simulink model "CEngDsT_VDDynTst"  (R2016b)
settings: configuration reference "CodeGenConfigSet" (kept outside this file)
values from neighbouring files (symbols this model uses):
  CEngDsT_dtMinDynTst_CUR = Calibration.Parameter    [init_CEngDsT_VDDynTst.m]
  CEngDsT_dtMinDynTst_CURX = Calibration.Parameter    [init_CEngDsT_VDDynTst.m]
  CEngDsT_nMinEnaAbsTst_C = Calibration.Parameter    [init_CEngDsT_VDDynTst.m]
  CEngDsT_nMinEnaDynTst_C = Calibration.Parameter    [init_CEngDsT_VDDynTst.m]
  CEngDsT_qMinAbsTst_C = Calibration.Parameter    [init_CEngDsT_VDDynTst.m]
  CEngDsT_qMinEnaDynTst_C = Calibration.Parameter    [init_CEngDsT_VDDynTst.m]
  CEngDsT_tiIniTmr_C = Calibration.Parameter    [init_CEngDsT_VDDynTst.m]
  CEngDsT_tiMaxAbsTst_CUR = Calibration.Parameter    [init_CEngDsT_VDDynTst.m]
  CEngDsT_tiMaxAbsTst_CURX = Calibration.Parameter    [init_CEngDsT_VDDynTst.m]
  CEngDsT_tiMaxDynTst_CUR = Calibration.Parameter    [init_CEngDsT_VDDynTst.m]
  CEngDsT_tiMaxDynTst_CURX = Calibration.Parameter    [init_CEngDsT_VDDynTst.m]
  CEngDsT_tMinAbsTst_CUR = Calibration.Parameter    [init_CEngDsT_VDDynTst.m]
  CEngDsT_tMinAbsTst_CURX = Calibration.Parameter    [init_CEngDsT_VDDynTst.m]
  CEngDsT_tMinThresDynTst_C = Calibration.Parameter    [init_CEngDsT_VDDynTst.m]
undefined symbols (not defined in the file or in its folder): CEngDsT_tTransf_CURX, CEngDsT_VDDynTst_DT, EngState_conv
libraries: CXLib x5
settings Model: Creator=lenovo  LastModifiedBy=wangrui
settings ConfigSetRef: SourceLocation=Base Workspace

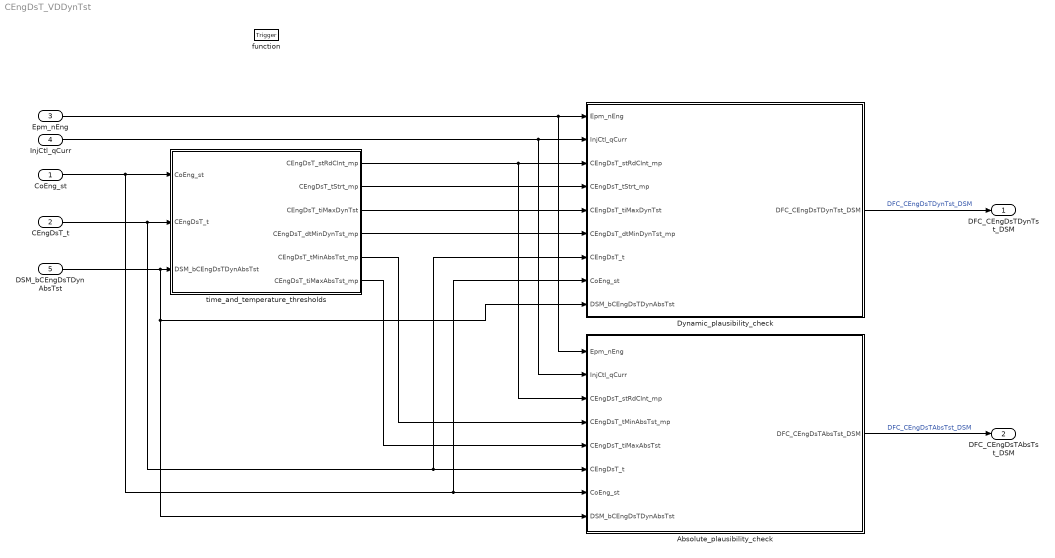
== system CEngDsT_VDDynTst ==
  CoEng_st : Inport  Description=Engine coordinator state  OutDataTypeStr=Enum: EngState_conv
  CEngDsT_t : Inport  Tag=deg  Description=engine coolant temperature after filter  Port=2  OutMin=-200  OutMax=200  OutDataTypeStr=Temp_deg
  Epm_nEng : Inport  Tag=rpm  Description=Engine speed  Port=3  OutMin=0  OutMax=6000  OutDataTypeStr=EngSpeed_rpm
  InjCtl_qCurr : Inport  Tag=mg/hub  Description=Torque generating engine fuel injection quantity  Port=4  OutMin=-319  OutMax=319  OutDataTypeStr=FuelMass_mg_hub
  DSM_bCEngDsTDynAbsTst : Inport  Description=state of FId_CEngDsTDynAbsTst  Port=5  OutMin=0  OutMax=1  OutDataTypeStr=boolean
  function : TriggerPort  TriggerType=function-call  VariantControl=Variant
  Absolute_plausibility_check : Subsystem  RequirementInfo={'other' 'CEngDsT_VDDynTst_requirements.doc' '@Simulink_requirement_item_3' 'true' '水温绝对值合理性校验' '' } %GIDa_49b2f334_2a18_42b0_a730_34b68f464cea
  Dynamic_plausibility_check : Subsystem  RequirementInfo={'other' 'CEngDsT_VDDynTst_requirements.doc' '@Simulink_requirement_item_2' 'true' '水温动态合理性校验' '' } %GIDa_29f8c977_1158_4d09_a78e_e4c79640a36b
  time_and_temperature_thresholds : Subsystem  RequirementInfo={'other' 'CEngDsT_VDDynTst_requirements.doc' '@Simulink_requirement_item_4' 'true' '水温动态和绝对值合理性校验参数计算' '' } %GIDa_436acdf0_f9c3_4326_aa51_de55f45c0a8d
  DFC_CEngDsTDynTst_DSM : Outport  Description=error state of DFC_CEngDsTDynTst  OutMin=0  OutMax=1  OutDataTypeStr=boolean
  DFC_CEngDsTAbsTst_DSM : Outport  Description=error state of DFC_CEngDsTAbsTst  Port=2  OutMin=0  OutMax=1  OutDataTypeStr=boolean
  wires:
  time_and_temperature_thresholds/3(CEngDsT_tiMaxDynTst) -> Dynamic_plausibility_check/5(CEngDsT_tiMaxDynTst)
  time_and_temperature_thresholds/6(CEngDsT_tiMaxAbsTst_mp) -> Absolute_plausibility_check/5(CEngDsT_tiMaxAbsTst)
  Epm_nEng/1 -> Absolute_plausibility_check/1(Epm_nEng), Dynamic_plausibility_check/1(Epm_nEng)
  time_and_temperature_thresholds/4(CEngDsT_dtMinDynTst_mp) -> Dynamic_plausibility_check/6(CEngDsT_dtMinDynTst_mp)
  time_and_temperature_thresholds/5(CEngDsT_tMinAbsTst_mp) -> Absolute_plausibility_check/4(CEngDsT_tMinAbsTst_mp)
  time_and_temperature_thresholds/1(CEngDsT_stRdClnt_mp) -> Absolute_plausibility_check/3(CEngDsT_stRdClnt_mp), Dynamic_plausibility_check/3(CEngDsT_stRdClnt_mp)
  InjCtl_qCurr/1 -> Absolute_plausibility_check/2(InjCtl_qCurr), Dynamic_plausibility_check/2(InjCtl_qCurr)
  time_and_temperature_thresholds/2(CEngDsT_tStrt_mp) -> Dynamic_plausibility_check/4(CEngDsT_tStrt_mp)
  CEngDsT_t/1 -> Dynamic_plausibility_check/7(CEngDsT_t), Absolute_plausibility_check/6(CEngDsT_t), time_and_temperature_thresholds/2(CEngDsT_t)
  CoEng_st/1 -> Dynamic_plausibility_check/8(CoEng_st), Absolute_plausibility_check/7(CoEng_st), time_and_temperature_thresholds/1(CoEng_st)
  DSM_bCEngDsTDynAbsTst/1 -> Absolute_plausibility_check/8(DSM_bCEngDsTDynAbsTst), Dynamic_plausibility_check/9(DSM_bCEngDsTDynAbsTst), time_and_temperature_thresholds/3(DSM_bCEngDsTDynAbsTst)
  Dynamic_plausibility_check/1(DFC_CEngDsTDynTst_DSM) -> DFC_CEngDsTDynTst_DSM/1  "DFC_CEngDsTDynTst_DSM"
  Absolute_plausibility_check/1(DFC_CEngDsTAbsTst_DSM) -> DFC_CEngDsTAbsTst_DSM/1  "DFC_CEngDsTAbsTst_DSM"

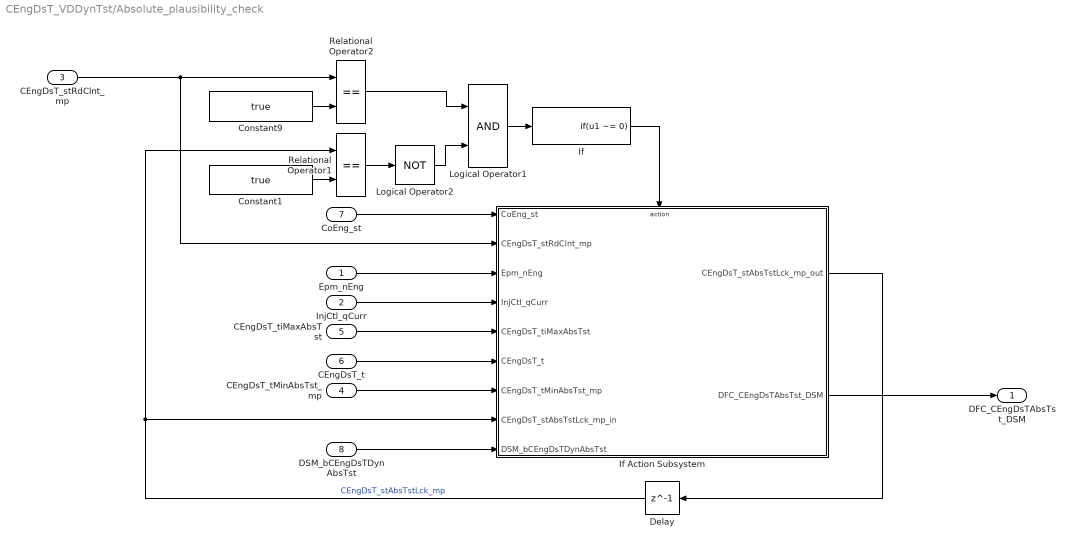
== system CEngDsT_VDDynTst/Absolute_plausibility_check ==
  Epm_nEng : Inport
  InjCtl_qCurr : Inport  Port=2
  CEngDsT_stRdClnt_mp : Inport  Port=3
  CEngDsT_tMinAbsTst_mp : Inport  Port=4
  CEngDsT_tiMaxAbsTst : Inport  Port=5
  CEngDsT_t : Inport  Port=6
  CoEng_st : Inport  Port=7
  DSM_bCEngDsTDynAbsTst : Inport  Description=state of FId_CEngDsTDynAbsTst  Port=8  OutMin=0  OutMax=1  OutDataTypeStr=boolean
  Constant1 : Constant  Value=true  VectorParams1D=off
  Constant9 : Constant  Value=true  VectorParams1D=off
  Delay : Delay  DelayLength=1  InitialCondition=0
  If : If  IfExpression=u1 ~= 0  ShowElse=off
  If Action Subsystem : Subsystem  TreatAsAtomicUnit=on
  Logical Operator1 : Logic  OutDataTypeStr=boolean
  Logical Operator2 : Logic  Operator=NOT  OutDataTypeStr=boolean
  Relational Operator1 : RelationalOperator  Operator===  OutDataTypeStr=boolean  RndMeth=Nearest  InputSameDT=on
  Relational Operator2 : RelationalOperator  Operator===  OutDataTypeStr=boolean  RndMeth=Nearest  InputSameDT=on
  DFC_CEngDsTAbsTst_DSM : Outport  Description=DFC_CEngDsTAbsTst  OutMin=0  OutMax=1  OutDataTypeStr=boolean
  wires:
  Delay/1 -> Relational Operator1/1, If Action Subsystem/8(CEngDsT_stAbsTstLck_mp_in)  "CEngDsT_stAbsTstLck_mp"
  If Action Subsystem/1(CEngDsT_stAbsTstLck_mp_out) -> Delay/1
  CEngDsT_stRdClnt_mp/1 -> If Action Subsystem/2(CEngDsT_stRdClnt_mp), Relational Operator2/1
  Constant9/1 -> Relational Operator2/2
  Constant1/1 -> Relational Operator1/2
  Relational Operator1/1 -> Logical Operator2/1
  Relational Operator2/1 -> Logical Operator1/1
  Logical Operator2/1 -> Logical Operator1/2
  Logical Operator1/1 -> If/1
  If/1 -> If Action Subsystem/Action
  CoEng_st/1 -> If Action Subsystem/1(CoEng_st)
  Epm_nEng/1 -> If Action Subsystem/3(Epm_nEng)
  InjCtl_qCurr/1 -> If Action Subsystem/4(InjCtl_qCurr)
  CEngDsT_tiMaxAbsTst/1 -> If Action Subsystem/5(CEngDsT_tiMaxAbsTst)
  CEngDsT_t/1 -> If Action Subsystem/6(CEngDsT_t)
  CEngDsT_tMinAbsTst_mp/1 -> If Action Subsystem/7(CEngDsT_tMinAbsTst_mp)
  DSM_bCEngDsTDynAbsTst/1 -> If Action Subsystem/9(DSM_bCEngDsTDynAbsTst)
  If Action Subsystem/2(DFC_CEngDsTAbsTst_DSM) -> DFC_CEngDsTAbsTst_DSM/1

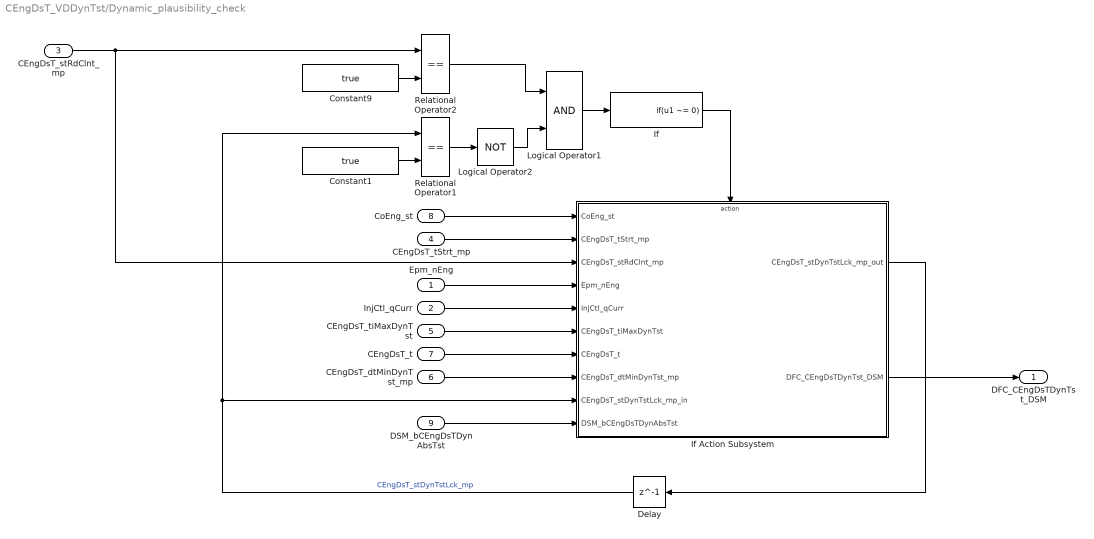
== system CEngDsT_VDDynTst/Dynamic_plausibility_check ==
  Epm_nEng : Inport
  InjCtl_qCurr : Inport  Port=2
  CEngDsT_stRdClnt_mp : Inport  Port=3
  CEngDsT_tStrt_mp : Inport  Port=4
  CEngDsT_tiMaxDynTst : Inport  Port=5
  CEngDsT_dtMinDynTst_mp : Inport  Port=6
  CEngDsT_t : Inport  Port=7
  CoEng_st : Inport  Port=8
  DSM_bCEngDsTDynAbsTst : Inport  Description=state of FId_CEngDsTDynAbsTst  Port=9  OutMin=0  OutMax=1  OutDataTypeStr=boolean
  Constant1 : Constant  Value=true  VectorParams1D=off
  Constant9 : Constant  Value=true  VectorParams1D=off
  Delay : Delay  DelayLength=1  InitialCondition=0
  If : If  IfExpression=u1 ~= 0  ShowElse=off
  If Action Subsystem : Subsystem  TreatAsAtomicUnit=on
  Logical Operator1 : Logic  OutDataTypeStr=boolean
  Logical Operator2 : Logic  Operator=NOT  OutDataTypeStr=boolean
  Relational Operator1 : RelationalOperator  Operator===  OutDataTypeStr=boolean  RndMeth=Nearest  InputSameDT=on
  Relational Operator2 : RelationalOperator  Operator===  OutDataTypeStr=boolean  RndMeth=Nearest  InputSameDT=on
  DFC_CEngDsTDynTst_DSM : Outport  Description=DFC_CEngDsTDynTst  OutMin=0  OutMax=1  OutDataTypeStr=boolean
  wires:
  CEngDsT_stRdClnt_mp/1 -> If Action Subsystem/3(CEngDsT_stRdClnt_mp), Relational Operator2/1
  Constant9/1 -> Relational Operator2/2
  Constant1/1 -> Relational Operator1/2
  Relational Operator1/1 -> Logical Operator2/1
  Relational Operator2/1 -> Logical Operator1/1
  Logical Operator2/1 -> Logical Operator1/2
  Logical Operator1/1 -> If/1
  If/1 -> If Action Subsystem/Action
  CEngDsT_tStrt_mp/1 -> If Action Subsystem/2(CEngDsT_tStrt_mp)
  CoEng_st/1 -> If Action Subsystem/1(CoEng_st)
  Epm_nEng/1 -> If Action Subsystem/4(Epm_nEng)
  InjCtl_qCurr/1 -> If Action Subsystem/5(InjCtl_qCurr)
  CEngDsT_tiMaxDynTst/1 -> If Action Subsystem/6(CEngDsT_tiMaxDynTst)
  CEngDsT_t/1 -> If Action Subsystem/7(CEngDsT_t)
  CEngDsT_dtMinDynTst_mp/1 -> If Action Subsystem/8(CEngDsT_dtMinDynTst_mp)
  If Action Subsystem/1(CEngDsT_stDynTstLck_mp_out) -> Delay/1
  Delay/1 -> If Action Subsystem/9(CEngDsT_stDynTstLck_mp_in), Relational Operator1/1  "CEngDsT_stDynTstLck_mp"
  DSM_bCEngDsTDynAbsTst/1 -> If Action Subsystem/10(DSM_bCEngDsTDynAbsTst)
  If Action Subsystem/2(DFC_CEngDsTDynTst_DSM) -> DFC_CEngDsTDynTst_DSM/1

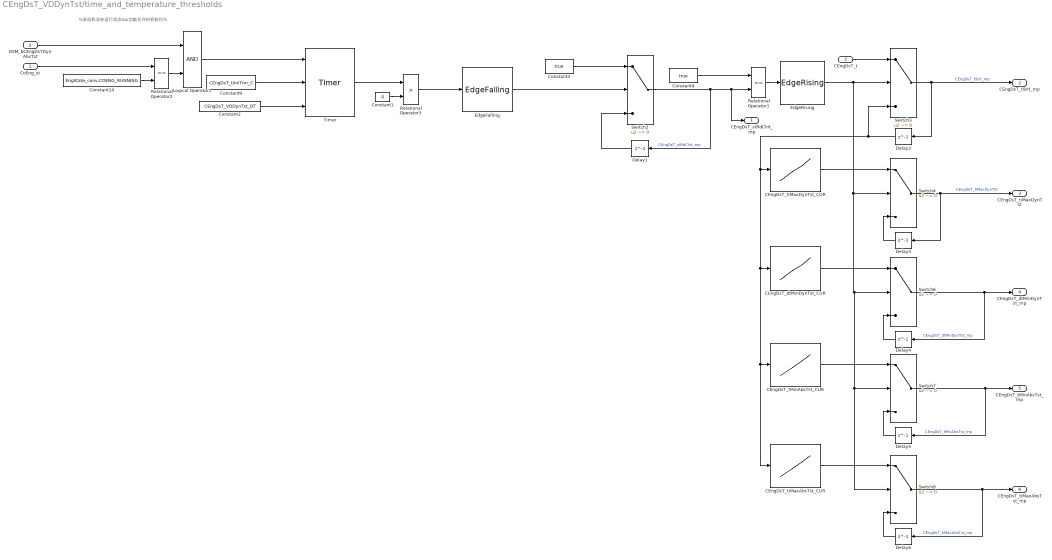
== system CEngDsT_VDDynTst/time_and_temperature_thresholds ==
  note: %发动机没在运行状态&&功能允许时初始化%
  CoEng_st : Inport
  CEngDsT_t : Inport  Port=2
  DSM_bCEngDsTDynAbsTst : Inport  Description=state of FId_CEngDsTDynAbsTst  Port=3  OutMin=0  OutMax=1  OutDataTypeStr=boolean
  CEngDsT_dtMinDynTst_CUR : Lookup_n-D  RequirementInfo={} %GIDa_f24a67d9_9be2_4f6a_98ff_fe8f3fd3d277  DialogController=Simulink.DDGSource  NumberOfTableDimensions=1  BreakpointsForDimension1=CEngDsT_dtMinDynTst_CURX  BreakpointsForDimension2=CEngDsT_tTransf_CURX  IndexSearchMethod=Linear search  BeginIndexSearchUsingPreviousIndexResult=on  Table=CEngDsT_dtMinDynTst_CUR  ExtrapMethod=Clip  UseLastTableValue=on  InternalRulePriority=Speed  OutDataTypeStr=Inherit: Inherit via back propagation  SaturateOnIntegerOverflow=on
  CEngDsT_tMinAbsTst_CUR : Lookup_n-D  RequirementInfo={} %GIDa_4fad5bf1_d5b2_4c41_9458_478ef92ce2f7  DialogController=Simulink.DDGSource  NumberOfTableDimensions=1  BreakpointsForDimension1=CEngDsT_tMinAbsTst_CURX  BreakpointsForDimension2=CEngDsT_tTransf_CURX  IndexSearchMethod=Linear search  BeginIndexSearchUsingPreviousIndexResult=on  Table=CEngDsT_tMinAbsTst_CUR  ExtrapMethod=Clip  UseLastTableValue=on  InternalRulePriority=Speed  OutDataTypeStr=Inherit: Inherit via back propagation  SaturateOnIntegerOverflow=on
  CEngDsT_tiMaxAbsTst_CUR : Lookup_n-D  RequirementInfo={} %GIDa_a4742909_2b6b_42c2_a6c4_82cb15b8cfec  DialogController=Simulink.DDGSource  NumberOfTableDimensions=1  BreakpointsForDimension1=CEngDsT_tiMaxAbsTst_CURX  BreakpointsForDimension2=CEngDsT_tTransf_CURX  IndexSearchMethod=Linear search  BeginIndexSearchUsingPreviousIndexResult=on  Table=CEngDsT_tiMaxAbsTst_CUR  ExtrapMethod=Clip  UseLastTableValue=on  InternalRulePriority=Speed  OutDataTypeStr=Inherit: Inherit via back propagation  SaturateOnIntegerOverflow=on
  CEngDsT_tiMaxDynTst_CUR : Lookup_n-D  RequirementInfo={} %GIDa_6227b4c9_a2a8_447e_8369_cb7c2ded31b1  DialogController=Simulink.DDGSource  NumberOfTableDimensions=1  BreakpointsForDimension1=CEngDsT_tiMaxDynTst_CURX  BreakpointsForDimension2=CEngDsT_tTransf_CURX  IndexSearchMethod=Linear search  BeginIndexSearchUsingPreviousIndexResult=on  Table=CEngDsT_tiMaxDynTst_CUR  ExtrapMethod=Clip  UseLastTableValue=on  InternalRulePriority=Speed  OutDataTypeStr=Inherit: Inherit via back propagation  SaturateOnIntegerOverflow=on
  Constant1 : Constant  Value=0  VectorParams1D=off  OutDataTypeStr=Inherit: Inherit via back propagation
  Constant14 : Constant  Value=EngState_conv.COENG_RUNNING
  Constant2 : Constant  Value=CEngDsT_VDDynTst_DT  VectorParams1D=off  OutDataTypeStr=Inherit: Inherit via back propagation
  Constant3 : Constant  Value=true  VectorParams1D=off  OutDataTypeStr=boolean
  Constant4 : Constant  Value=true  VectorParams1D=off  OutDataTypeStr=boolean
  Constant9 : Constant  Value=CEngDsT_tiIniTmr_C  VectorParams1D=off
  Delay{1..6} (6 alike) : Delay  DialogController=Simulink.DDGSource  DelayLength=1  InitialCondition=0
  EdgeFalling : CXLib/EdgeFalling
  EdgeRising : CXLib/EdgeRising
  Logical Operator1 : Logic  OutDataTypeStr=boolean
  Relational Operator1 : RelationalOperator  Operator===  OutDataTypeStr=boolean  RndMeth=Nearest  InputSameDT=on
  Relational Operator2 : RelationalOperator  Operator===  OutDataTypeStr=boolean  RndMeth=Nearest  InputSameDT=on
  Relational Operator3 : RelationalOperator  Operator=>  OutDataTypeStr=boolean  RndMeth=Nearest  InputSameDT=on
  Switch{2..4,6..8} (6 alike) : Switch  Criteria=u2 ~= 0  InputSameDT=on
  Timer : CXLib/Timer
  CEngDsT_stRdClnt_mp : Outport
  CEngDsT_tStrt_mp : Outport  Port=2
  CEngDsT_tiMaxDynTst : Outport  Port=3
  CEngDsT_dtMinDynTst_mp : Outport  Port=4
  CEngDsT_tMinAbsTst_mp : Outport  Port=5
  CEngDsT_tiMaxAbsTst_mp : Outport  Port=6
  wires:
  Constant2/1 -> Timer/3
  Relational Operator3/1 -> EdgeFalling/1
  Constant1/1 -> Relational Operator3/2
  Timer/1 -> Relational Operator3/1
  Constant9/1 -> Timer/2
  CEngDsT_tiMaxDynTst_CUR/1 -> Switch4/1
  Delay2/1 -> Switch3/3, CEngDsT_tiMaxAbsTst_CUR/1, CEngDsT_tMinAbsTst_CUR/1, CEngDsT_dtMinDynTst_CUR/1, CEngDsT_tiMaxDynTst_CUR/1
  Switch3/1 -> CEngDsT_tStrt_mp/1, Delay2/1  "CEngDsT_tStrt_mp"
  CEngDsT_t/1 -> Switch3/1
  EdgeRising/1 -> Switch3/2, Switch4/2, Switch6/2, Switch7/2, Switch8/2
  Relational Operator1/1 -> EdgeRising/1
  Constant4/1 -> Relational Operator1/1
  Delay1/1 -> Switch2/3
  Switch2/1 -> Delay1/1, Relational Operator1/2, CEngDsT_stRdClnt_mp/1  "CEngDsT_stRdClnt_mp"
  Constant3/1 -> Switch2/1
  EdgeFalling/1 -> Switch2/2
  Logical Operator1/1 -> Timer/1
  Relational Operator2/1 -> Logical Operator1/2
  DSM_bCEngDsTDynAbsTst/1 -> Logical Operator1/1
  CoEng_st/1 -> Relational Operator2/1
  Constant14/1 -> Relational Operator2/2
  Delay3/1 -> Switch4/3
  CEngDsT_tiMaxAbsTst_CUR/1 -> Switch8/1
  CEngDsT_tMinAbsTst_CUR/1 -> Switch7/1
  Switch7/1 -> CEngDsT_tMinAbsTst_mp/1, Delay5/1  "CEngDsT_tMinAbsTst_mp"
  Delay6/1 -> Switch8/3
  Delay5/1 -> Switch7/3
  Delay4/1 -> Switch6/3
  Switch8/1 -> Delay6/1, CEngDsT_tiMaxAbsTst_mp/1  "CEngDsT_tiMaxAbsTst_mp"
  CEngDsT_dtMinDynTst_CUR/1 -> Switch6/1
  Switch6/1 -> Delay4/1, CEngDsT_dtMinDynTst_mp/1  "CEngDsT_dtMinDynTst_mp"
  Switch4/1 -> Delay3/1, CEngDsT_tiMaxDynTst/1  "CEngDsT_tiMaxDynTst"

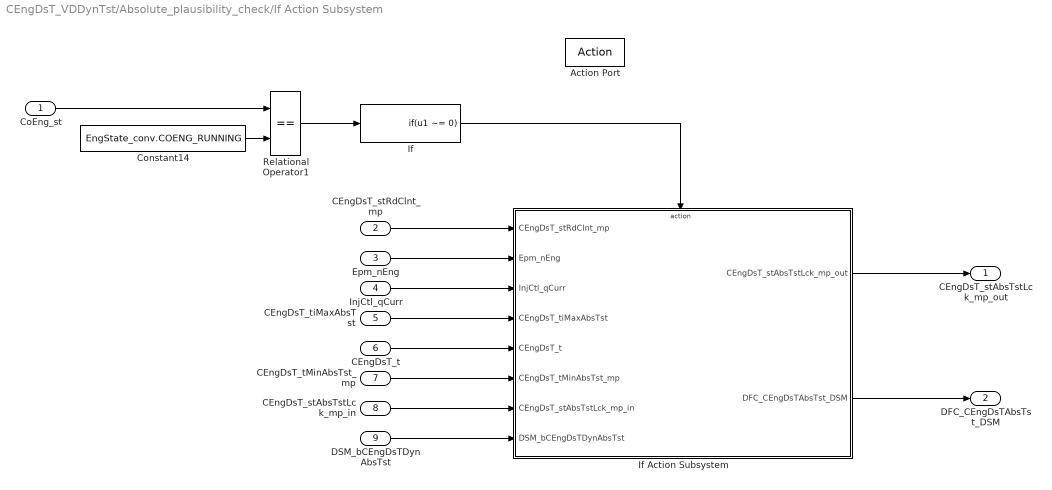
== system CEngDsT_VDDynTst/Absolute_plausibility_check/If Action Subsystem ==
  CoEng_st : Inport
  CEngDsT_stRdClnt_mp : Inport  Port=2
  Epm_nEng : Inport  Port=3
  InjCtl_qCurr : Inport  Port=4
  CEngDsT_tiMaxAbsTst : Inport  Port=5
  CEngDsT_t : Inport  Port=6
  CEngDsT_tMinAbsTst_mp : Inport  Port=7
  CEngDsT_stAbsTstLck_mp_in : Inport  Port=8
  DSM_bCEngDsTDynAbsTst : Inport  Description=state of FId_CEngDsTDynAbsTst  Port=9  OutMin=0  OutMax=1  OutDataTypeStr=boolean
  Action Port : ActionPort
  Constant14 : Constant  Value=EngState_conv.COENG_RUNNING
  If : If  IfExpression=u1 ~= 0  ShowElse=off
  If Action Subsystem : Subsystem  TreatAsAtomicUnit=on
  Relational Operator1 : RelationalOperator  Operator===  OutDataTypeStr=boolean  RndMeth=Nearest  InputSameDT=on
  CEngDsT_stAbsTstLck_mp_out : Outport
  DFC_CEngDsTAbsTst_DSM : Outport  Description=DFC_CEngDsTAbsTst  Port=2  OutMin=0  OutMax=1  OutDataTypeStr=boolean
  wires:
  If/1 -> If Action Subsystem/Action
  CoEng_st/1 -> Relational Operator1/1
  Constant14/1 -> Relational Operator1/2
  Relational Operator1/1 -> If/1
  If Action Subsystem/1(CEngDsT_stAbsTstLck_mp_out) -> CEngDsT_stAbsTstLck_mp_out/1
  CEngDsT_stRdClnt_mp/1 -> If Action Subsystem/1(CEngDsT_stRdClnt_mp)
  Epm_nEng/1 -> If Action Subsystem/2(Epm_nEng)
  InjCtl_qCurr/1 -> If Action Subsystem/3(InjCtl_qCurr)
  CEngDsT_tiMaxAbsTst/1 -> If Action Subsystem/4(CEngDsT_tiMaxAbsTst)
  CEngDsT_t/1 -> If Action Subsystem/5(CEngDsT_t)
  CEngDsT_tMinAbsTst_mp/1 -> If Action Subsystem/6(CEngDsT_tMinAbsTst_mp)
  CEngDsT_stAbsTstLck_mp_in/1 -> If Action Subsystem/7(CEngDsT_stAbsTstLck_mp_in)
  DSM_bCEngDsTDynAbsTst/1 -> If Action Subsystem/8(DSM_bCEngDsTDynAbsTst)
  If Action Subsystem/2(DFC_CEngDsTAbsTst_DSM) -> DFC_CEngDsTAbsTst_DSM/1

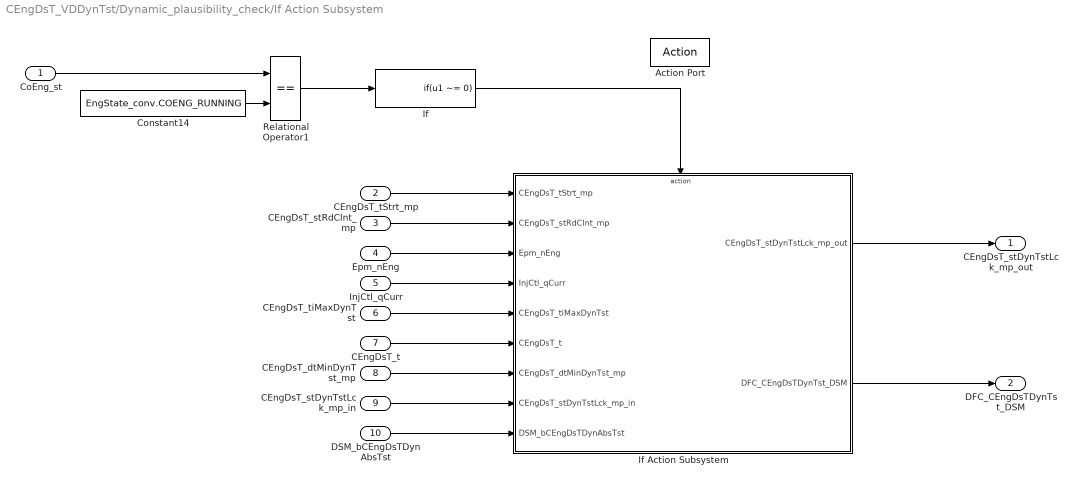
== system CEngDsT_VDDynTst/Dynamic_plausibility_check/If Action Subsystem ==
  CoEng_st : Inport
  CEngDsT_tStrt_mp : Inport  Port=2
  CEngDsT_stRdClnt_mp : Inport  Port=3
  Epm_nEng : Inport  Port=4
  InjCtl_qCurr : Inport  Port=5
  CEngDsT_tiMaxDynTst : Inport  Port=6
  CEngDsT_t : Inport  Port=7
  CEngDsT_dtMinDynTst_mp : Inport  Port=8
  CEngDsT_stDynTstLck_mp_in : Inport  Port=9
  DSM_bCEngDsTDynAbsTst : Inport  Description=state of FId_CEngDsTDynAbsTst  Port=10  OutMin=0  OutMax=1  OutDataTypeStr=boolean
  Action Port : ActionPort
  Constant14 : Constant  Value=EngState_conv.COENG_RUNNING
  If : If  IfExpression=u1 ~= 0  ShowElse=off
  If Action Subsystem : Subsystem  TreatAsAtomicUnit=on
  Relational Operator1 : RelationalOperator  Operator===  OutDataTypeStr=boolean  RndMeth=Nearest  InputSameDT=on
  CEngDsT_stDynTstLck_mp_out : Outport
  DFC_CEngDsTDynTst_DSM : Outport  Description=DFC_CEngDsTDynTst  Port=2  OutMin=0  OutMax=1  OutDataTypeStr=boolean
  wires:
  If/1 -> If Action Subsystem/Action
  CoEng_st/1 -> Relational Operator1/1
  Constant14/1 -> Relational Operator1/2
  Relational Operator1/1 -> If/1
  If Action Subsystem/1(CEngDsT_stDynTstLck_mp_out) -> CEngDsT_stDynTstLck_mp_out/1
  CEngDsT_stRdClnt_mp/1 -> If Action Subsystem/2(CEngDsT_stRdClnt_mp)
  Epm_nEng/1 -> If Action Subsystem/3(Epm_nEng)
  InjCtl_qCurr/1 -> If Action Subsystem/4(InjCtl_qCurr)
  CEngDsT_tStrt_mp/1 -> If Action Subsystem/1(CEngDsT_tStrt_mp)
  CEngDsT_tiMaxDynTst/1 -> If Action Subsystem/5(CEngDsT_tiMaxDynTst)
  CEngDsT_t/1 -> If Action Subsystem/6(CEngDsT_t)
  CEngDsT_dtMinDynTst_mp/1 -> If Action Subsystem/7(CEngDsT_dtMinDynTst_mp)
  CEngDsT_stDynTstLck_mp_in/1 -> If Action Subsystem/8(CEngDsT_stDynTstLck_mp_in)
  DSM_bCEngDsTDynAbsTst/1 -> If Action Subsystem/9(DSM_bCEngDsTDynAbsTst)
  If Action Subsystem/2(DFC_CEngDsTDynTst_DSM) -> DFC_CEngDsTDynTst_DSM/1

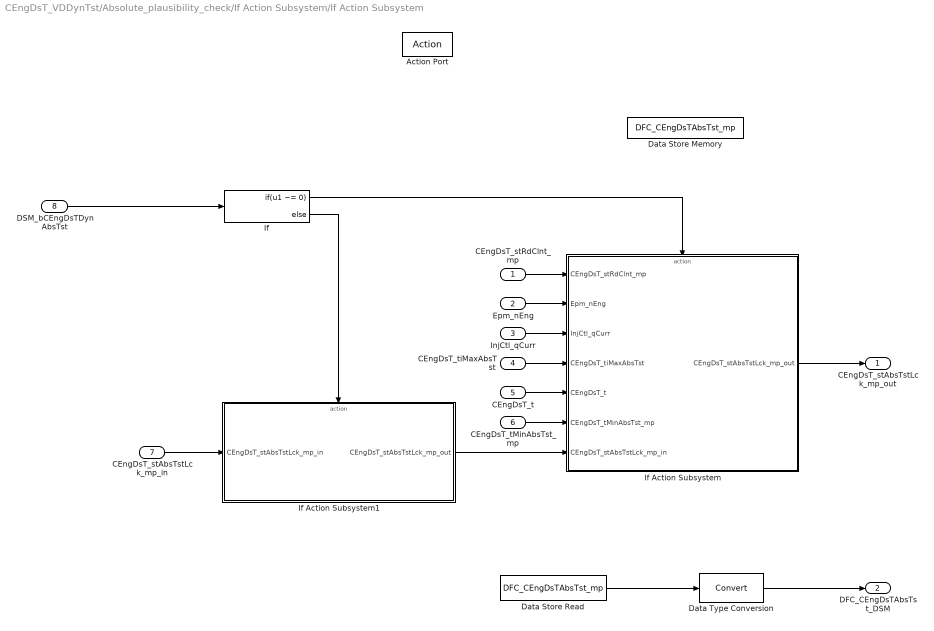
== system CEngDsT_VDDynTst/Absolute_plausibility_check/If Action Subsystem/If Action Subsystem ==
  CEngDsT_stRdClnt_mp : Inport
  Epm_nEng : Inport  Port=2
  InjCtl_qCurr : Inport  Port=3
  CEngDsT_tiMaxAbsTst : Inport  Port=4
  CEngDsT_t : Inport  Port=5
  CEngDsT_tMinAbsTst_mp : Inport  Port=6
  CEngDsT_stAbsTstLck_mp_in : Inport  Port=7
  DSM_bCEngDsTDynAbsTst : Inport  Description=state of FId_CEngDsTDynAbsTst  Port=8  OutMin=0  OutMax=1  OutDataTypeStr=boolean
  Action Port : ActionPort
  Data Store Memory : DataStoreMemory  DataStoreName=DFC_CEngDsTAbsTst_mp  ReadBeforeWriteMsg=warning  WriteAfterWriteMsg=warning  WriteAfterReadMsg=warning  ShowAdditionalParam=off
  Data Store Read : DataStoreRead  DataStoreName=DFC_CEngDsTAbsTst_mp
  Data Type Conversion : DataTypeConversion
  If : If  IfExpression=u1 ~= 0
  If Action Subsystem : Subsystem  TreatAsAtomicUnit=on
  If Action Subsystem1 : Subsystem  TreatAsAtomicUnit=on
  CEngDsT_stAbsTstLck_mp_out : Outport
  DFC_CEngDsTAbsTst_DSM : Outport  Description=DFC_CEngDsTAbsTst  Port=2  OutMin=0  OutMax=1  OutDataTypeStr=boolean
  wires:
  DSM_bCEngDsTDynAbsTst/1 -> If/1
  If/1 -> If Action Subsystem/Action
  If/2 -> If Action Subsystem1/Action
  If Action Subsystem1/1(CEngDsT_stAbsTstLck_mp_out) -> If Action Subsystem/7(CEngDsT_stAbsTstLck_mp_in)
  CEngDsT_stRdClnt_mp/1 -> If Action Subsystem/1(CEngDsT_stRdClnt_mp)
  If Action Subsystem/1(CEngDsT_stAbsTstLck_mp_out) -> CEngDsT_stAbsTstLck_mp_out/1
  CEngDsT_stAbsTstLck_mp_in/1 -> If Action Subsystem1/1(CEngDsT_stAbsTstLck_mp_in)
  Epm_nEng/1 -> If Action Subsystem/2(Epm_nEng)
  CEngDsT_tiMaxAbsTst/1 -> If Action Subsystem/4(CEngDsT_tiMaxAbsTst)
  InjCtl_qCurr/1 -> If Action Subsystem/3(InjCtl_qCurr)
  CEngDsT_t/1 -> If Action Subsystem/5(CEngDsT_t)
  CEngDsT_tMinAbsTst_mp/1 -> If Action Subsystem/6(CEngDsT_tMinAbsTst_mp)
  Data Store Read/1 -> Data Type Conversion/1
  Data Type Conversion/1 -> DFC_CEngDsTAbsTst_DSM/1

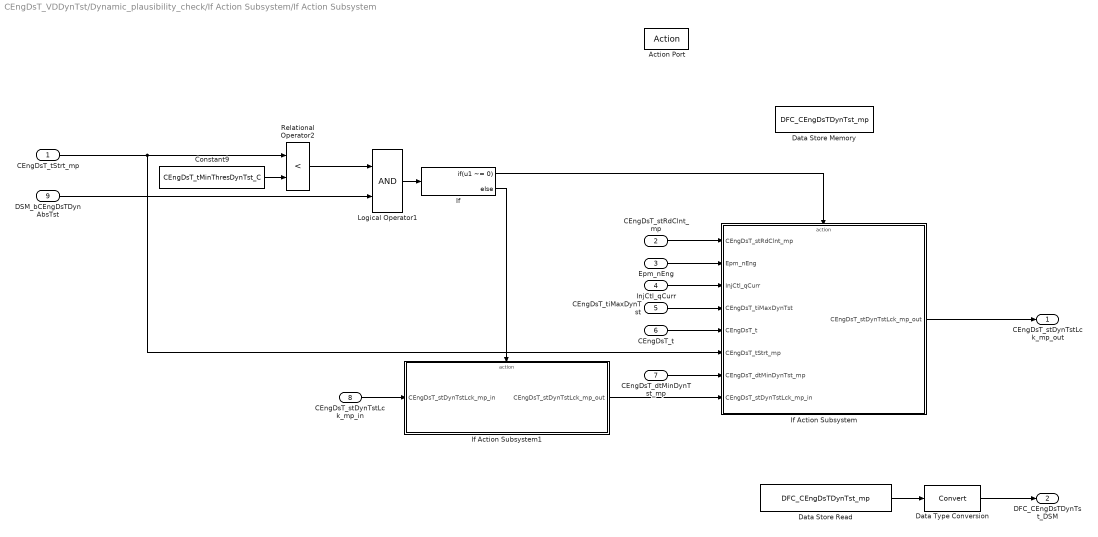
== system CEngDsT_VDDynTst/Dynamic_plausibility_check/If Action Subsystem/If Action Subsystem ==
  CEngDsT_tStrt_mp : Inport
  CEngDsT_stRdClnt_mp : Inport  Port=2
  Epm_nEng : Inport  Port=3
  InjCtl_qCurr : Inport  Port=4
  CEngDsT_tiMaxDynTst : Inport  Port=5
  CEngDsT_t : Inport  Port=6
  CEngDsT_dtMinDynTst_mp : Inport  Port=7
  CEngDsT_stDynTstLck_mp_in : Inport  Port=8
  DSM_bCEngDsTDynAbsTst : Inport  Description=state of FId_CEngDsTDynAbsTst  Port=9  OutMin=0  OutMax=1  OutDataTypeStr=boolean
  Action Port : ActionPort
  Constant9 : Constant  Value=CEngDsT_tMinThresDynTst_C  VectorParams1D=off
  Data Store Memory : DataStoreMemory  DataStoreName=DFC_CEngDsTDynTst_mp  ReadBeforeWriteMsg=warning  WriteAfterWriteMsg=warning  WriteAfterReadMsg=warning  ShowAdditionalParam=off
  Data Store Read : DataStoreRead  DataStoreName=DFC_CEngDsTDynTst_mp
  Data Type Conversion : DataTypeConversion
  If : If  IfExpression=u1 ~= 0
  If Action Subsystem : Subsystem  TreatAsAtomicUnit=on
  If Action Subsystem1 : Subsystem  TreatAsAtomicUnit=on
  Logical Operator1 : Logic  OutDataTypeStr=boolean
  Relational Operator2 : RelationalOperator  Operator=<  OutDataTypeStr=boolean  RndMeth=Nearest  InputSameDT=on
  CEngDsT_stDynTstLck_mp_out : Outport
  DFC_CEngDsTDynTst_DSM : Outport  Description=DFC_CEngDsTDynTst  Port=2  OutMin=0  OutMax=1  OutDataTypeStr=boolean
  wires:
  Constant9/1 -> Relational Operator2/2
  Relational Operator2/1 -> Logical Operator1/1
  Logical Operator1/1 -> If/1
  DSM_bCEngDsTDynAbsTst/1 -> Logical Operator1/2
  If/1 -> If Action Subsystem/Action
  If/2 -> If Action Subsystem1/Action
  If Action Subsystem1/1(CEngDsT_stDynTstLck_mp_out) -> If Action Subsystem/8(CEngDsT_stDynTstLck_mp_in)
  CEngDsT_stRdClnt_mp/1 -> If Action Subsystem/1(CEngDsT_stRdClnt_mp)
  If Action Subsystem/1(CEngDsT_stDynTstLck_mp_out) -> CEngDsT_stDynTstLck_mp_out/1
  CEngDsT_stDynTstLck_mp_in/1 -> If Action Subsystem1/1(CEngDsT_stDynTstLck_mp_in)
  Epm_nEng/1 -> If Action Subsystem/2(Epm_nEng)
  CEngDsT_tiMaxDynTst/1 -> If Action Subsystem/4(CEngDsT_tiMaxDynTst)
  InjCtl_qCurr/1 -> If Action Subsystem/3(InjCtl_qCurr)
  CEngDsT_t/1 -> If Action Subsystem/5(CEngDsT_t)
  CEngDsT_tStrt_mp/1 -> If Action Subsystem/6(CEngDsT_tStrt_mp), Relational Operator2/1
  CEngDsT_dtMinDynTst_mp/1 -> If Action Subsystem/7(CEngDsT_dtMinDynTst_mp)
  Data Store Read/1 -> Data Type Conversion/1
  Data Type Conversion/1 -> DFC_CEngDsTDynTst_DSM/1

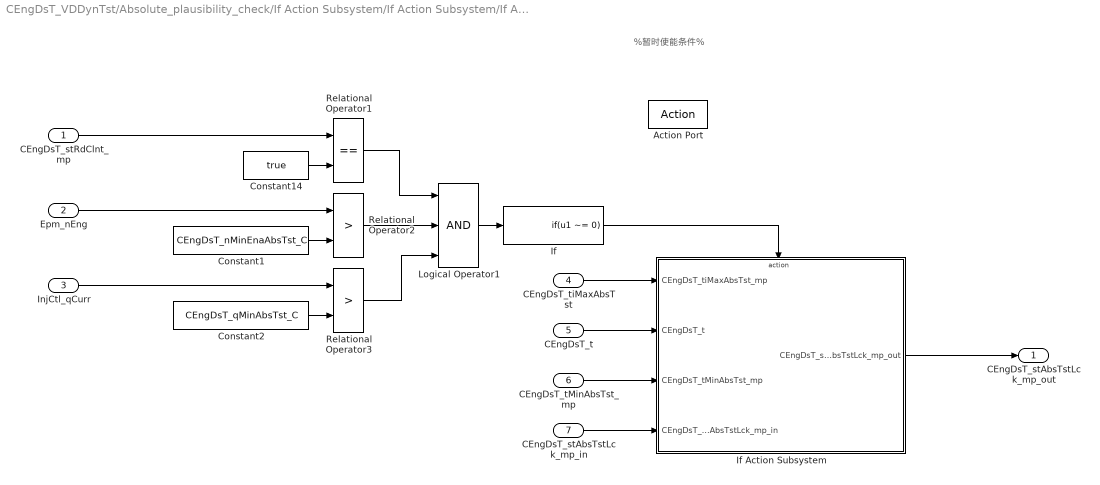
== system CEngDsT_VDDynTst/Absolute_plausibility_check/If Action Subsystem/If Action Subsystem/If Action Subsystem ==
  note: %暂时使能条件%
  CEngDsT_stRdClnt_mp : Inport
  Epm_nEng : Inport  Port=2
  InjCtl_qCurr : Inport  Port=3
  CEngDsT_tiMaxAbsTst : Inport  Port=4
  CEngDsT_t : Inport  Port=5
  CEngDsT_tMinAbsTst_mp : Inport  Port=6
  CEngDsT_stAbsTstLck_mp_in : Inport  Port=7
  Action Port : ActionPort
  Constant1 : Constant  Value=CEngDsT_nMinEnaAbsTst_C  OutDataTypeStr=Inherit: Inherit via back propagation
  Constant14 : Constant  Value=true  OutDataTypeStr=Inherit: Inherit via back propagation
  Constant2 : Constant  Value=CEngDsT_qMinAbsTst_C  OutDataTypeStr=Inherit: Inherit via back propagation
  If : If  IfExpression=u1 ~= 0  ShowElse=off
  If Action Subsystem : Subsystem  TreatAsAtomicUnit=on
  Logical Operator1 : Logic  Inputs=3  OutDataTypeStr=boolean
  Relational Operator1 : RelationalOperator  Operator===  OutDataTypeStr=boolean  RndMeth=Nearest  InputSameDT=on
  Relational Operator2 : RelationalOperator  Operator=>  OutDataTypeStr=boolean  RndMeth=Nearest  InputSameDT=on
  Relational Operator3 : RelationalOperator  Operator=>  OutDataTypeStr=boolean  RndMeth=Nearest  InputSameDT=on
  CEngDsT_stAbsTstLck_mp_out : Outport
  wires:
  If/1 -> If Action Subsystem/Action
  Constant14/1 -> Relational Operator1/2
  Relational Operator1/1 -> Logical Operator1/1
  Epm_nEng/1 -> Relational Operator2/1
  Constant1/1 -> Relational Operator2/2
  InjCtl_qCurr/1 -> Relational Operator3/1
  Constant2/1 -> Relational Operator3/2
  Logical Operator1/1 -> If/1
  Relational Operator2/1 -> Logical Operator1/2
  Relational Operator3/1 -> Logical Operator1/3
  If Action Subsystem/1(CEngDsT_stAbsTstLck_mp_out) -> CEngDsT_stAbsTstLck_mp_out/1
  CEngDsT_tiMaxAbsTst/1 -> If Action Subsystem/1(CEngDsT_tiMaxAbsTst_mp)
  CEngDsT_t/1 -> If Action Subsystem/2(CEngDsT_t)
  CEngDsT_stRdClnt_mp/1 -> Relational Operator1/1
  CEngDsT_tMinAbsTst_mp/1 -> If Action Subsystem/3(CEngDsT_tMinAbsTst_mp)
  CEngDsT_stAbsTstLck_mp_in/1 -> If Action Subsystem/4(CEngDsT_stAbsTstLck_mp_in)

== system CEngDsT_VDDynTst/Absolute_plausibility_check/If Action Subsystem/If Action Subsystem/If Action Subsystem1 ==
  CEngDsT_stAbsTstLck_mp_in : Inport
  Action Port : ActionPort
  Constant1 : Constant  OutDataTypeStr=boolean
  Constant3 : Constant  Value=true  OutDataTypeStr=Inherit: Inherit via back propagation
  Switch1 : Switch  Criteria=u2 ~= 0  InputSameDT=on
  CEngDsT_stAbsTstLck_mp_out : Outport
  wires:
  Constant3/1 -> Switch1/1
  CEngDsT_stAbsTstLck_mp_in/1 -> Switch1/3
  Switch1/1 -> CEngDsT_stAbsTstLck_mp_out/1
  Constant1/1 -> Switch1/2

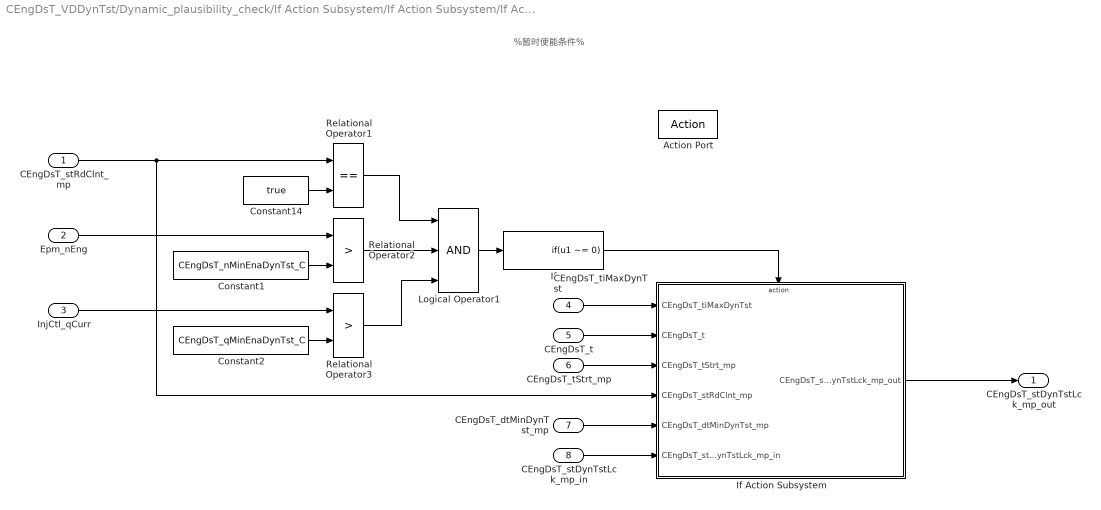
== system CEngDsT_VDDynTst/Dynamic_plausibility_check/If Action Subsystem/If Action Subsystem/If Action Subsystem ==
  note: %暂时使能条件%
  CEngDsT_stRdClnt_mp : Inport
  Epm_nEng : Inport  Port=2
  InjCtl_qCurr : Inport  Port=3
  CEngDsT_tiMaxDynTst : Inport  Port=4
  CEngDsT_t : Inport  Port=5
  CEngDsT_tStrt_mp : Inport  Port=6
  CEngDsT_dtMinDynTst_mp : Inport  Port=7
  CEngDsT_stDynTstLck_mp_in : Inport  Port=8
  Action Port : ActionPort
  Constant1 : Constant  Value=CEngDsT_nMinEnaDynTst_C  OutDataTypeStr=Inherit: Inherit via back propagation
  Constant14 : Constant  Value=true  OutDataTypeStr=Inherit: Inherit via back propagation
  Constant2 : Constant  Value=CEngDsT_qMinEnaDynTst_C  OutDataTypeStr=Inherit: Inherit via back propagation
  If : If  IfExpression=u1 ~= 0  ShowElse=off
  If Action Subsystem : Subsystem  TreatAsAtomicUnit=on
  Logical Operator1 : Logic  Inputs=3  OutDataTypeStr=boolean
  Relational Operator1 : RelationalOperator  Operator===  OutDataTypeStr=boolean  RndMeth=Nearest  InputSameDT=on
  Relational Operator2 : RelationalOperator  Operator=>  OutDataTypeStr=boolean  RndMeth=Nearest  InputSameDT=on
  Relational Operator3 : RelationalOperator  Operator=>  OutDataTypeStr=boolean  RndMeth=Nearest  InputSameDT=on
  CEngDsT_stDynTstLck_mp_out : Outport
  wires:
  If/1 -> If Action Subsystem/Action
  Constant14/1 -> Relational Operator1/2
  Relational Operator1/1 -> Logical Operator1/1
  Epm_nEng/1 -> Relational Operator2/1
  Constant1/1 -> Relational Operator2/2
  InjCtl_qCurr/1 -> Relational Operator3/1
  Constant2/1 -> Relational Operator3/2
  Logical Operator1/1 -> If/1
  Relational Operator2/1 -> Logical Operator1/2
  Relational Operator3/1 -> Logical Operator1/3
  If Action Subsystem/1(CEngDsT_stDynTstLck_mp_out) -> CEngDsT_stDynTstLck_mp_out/1
  CEngDsT_tiMaxDynTst/1 -> If Action Subsystem/1(CEngDsT_tiMaxDynTst)
  CEngDsT_t/1 -> If Action Subsystem/2(CEngDsT_t)
  CEngDsT_tStrt_mp/1 -> If Action Subsystem/3(CEngDsT_tStrt_mp)
  CEngDsT_stRdClnt_mp/1 -> Relational Operator1/1, If Action Subsystem/4(CEngDsT_stRdClnt_mp)
  CEngDsT_dtMinDynTst_mp/1 -> If Action Subsystem/5(CEngDsT_dtMinDynTst_mp)
  CEngDsT_stDynTstLck_mp_in/1 -> If Action Subsystem/6(CEngDsT_stDynTstLck_mp_in)

== system CEngDsT_VDDynTst/Dynamic_plausibility_check/If Action Subsystem/If Action Subsystem/If Action Subsystem1 ==
  CEngDsT_stDynTstLck_mp_in : Inport
  Action Port : ActionPort
  Constant1 : Constant  OutDataTypeStr=boolean
  Constant3 : Constant  Value=true  OutDataTypeStr=Inherit: Inherit via back propagation
  Switch1 : Switch  Criteria=u2 ~= 0  InputSameDT=on
  CEngDsT_stDynTstLck_mp_out : Outport
  wires:
  Constant3/1 -> Switch1/1
  CEngDsT_stDynTstLck_mp_in/1 -> Switch1/3
  Switch1/1 -> CEngDsT_stDynTstLck_mp_out/1
  Constant1/1 -> Switch1/2

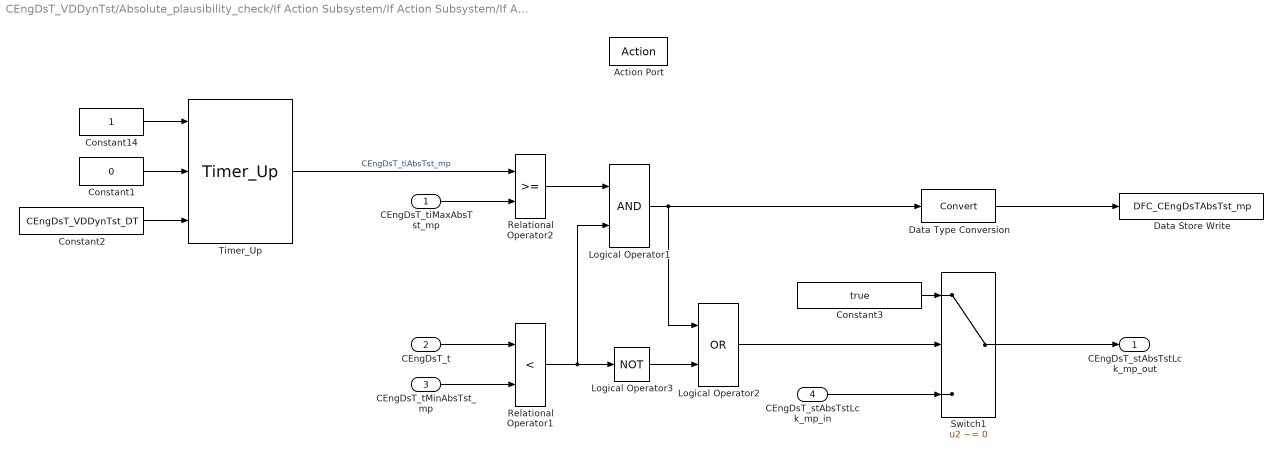
== system CEngDsT_VDDynTst/Absolute_plausibility_check/If Action Subsystem/If Action Subsystem/If Action Subsystem/If Action Subsystem ==
  CEngDsT_tiMaxAbsTst_mp : Inport
  CEngDsT_t : Inport  Port=2
  CEngDsT_tMinAbsTst_mp : Inport  Port=3
  CEngDsT_stAbsTstLck_mp_in : Inport  Port=4
  Action Port : ActionPort
  Constant1 : Constant  Value=0  OutDataTypeStr=boolean
  Constant14 : Constant  OutDataTypeStr=boolean
  Constant2 : Constant  Value=CEngDsT_VDDynTst_DT  OutDataTypeStr=Inherit: Inherit via back propagation
  Constant3 : Constant  Value=true  OutDataTypeStr=Inherit: Inherit via back propagation
  Data Store Write : DataStoreWrite  DataStoreName=DFC_CEngDsTAbsTst_mp
  Data Type Conversion : DataTypeConversion
  Logical Operator1 : Logic  OutDataTypeStr=boolean
  Logical Operator2 : Logic  Operator=OR  OutDataTypeStr=boolean
  Logical Operator3 : Logic  Operator=NOT  OutDataTypeStr=boolean
  Relational Operator1 : RelationalOperator  Operator=<  OutDataTypeStr=boolean  RndMeth=Nearest  InputSameDT=on
  Relational Operator2 : RelationalOperator  OutDataTypeStr=boolean  RndMeth=Nearest  InputSameDT=on
  Switch1 : Switch  Criteria=u2 ~= 0  InputSameDT=on
  Timer_Up : CXLib/Timer_Up
  CEngDsT_stAbsTstLck_mp_out : Outport
  wires:
  Constant2/1 -> Timer_Up/3
  Timer_Up/1 -> Relational Operator2/1  "CEngDsT_tiAbsTst_mp"
  Constant14/1 -> Timer_Up/1
  Constant1/1 -> Timer_Up/2
  CEngDsT_tiMaxAbsTst_mp/1 -> Relational Operator2/2
  Relational Operator2/1 -> Logical Operator1/1
  CEngDsT_t/1 -> Relational Operator1/1
  CEngDsT_tMinAbsTst_mp/1 -> Relational Operator1/2
  Relational Operator1/1 -> Logical Operator3/1, Logical Operator1/2
  Logical Operator3/1 -> Logical Operator2/2
  Switch1/1 -> CEngDsT_stAbsTstLck_mp_out/1
  Logical Operator1/1 -> Data Type Conversion/1, Logical Operator2/1
  Logical Operator2/1 -> Switch1/2
  Constant3/1 -> Switch1/1
  CEngDsT_stAbsTstLck_mp_in/1 -> Switch1/3
  Data Type Conversion/1 -> Data Store Write/1

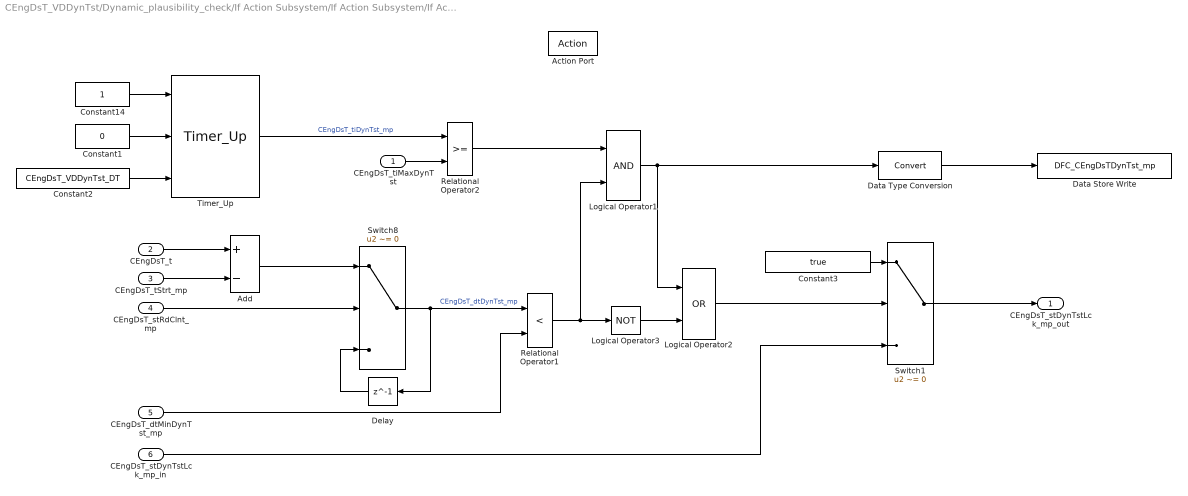
== system CEngDsT_VDDynTst/Dynamic_plausibility_check/If Action Subsystem/If Action Subsystem/If Action Subsystem/If Action Subsystem ==
  CEngDsT_tiMaxDynTst : Inport
  CEngDsT_t : Inport  Port=2
  CEngDsT_tStrt_mp : Inport  Port=3
  CEngDsT_stRdClnt_mp : Inport  Port=4
  CEngDsT_dtMinDynTst_mp : Inport  Port=5
  CEngDsT_stDynTstLck_mp_in : Inport  Port=6
  Action Port : ActionPort
  Add : Sum  Inputs=+-  OutDataTypeStr=Inherit: Inherit via back propagation  SaturateOnIntegerOverflow=on  InputSameDT=on
  Constant1 : Constant  Value=0  OutDataTypeStr=boolean
  Constant14 : Constant  OutDataTypeStr=boolean
  Constant2 : Constant  Value=CEngDsT_VDDynTst_DT  OutDataTypeStr=Inherit: Inherit via back propagation
  Constant3 : Constant  Value=true  OutDataTypeStr=Inherit: Inherit via back propagation
  Data Store Write : DataStoreWrite  DataStoreName=DFC_CEngDsTDynTst_mp
  Data Type Conversion : DataTypeConversion
  Delay : Delay  DelayLength=1  InitialCondition=0
  Logical Operator1 : Logic  OutDataTypeStr=boolean
  Logical Operator2 : Logic  Operator=OR  OutDataTypeStr=boolean
  Logical Operator3 : Logic  Operator=NOT  OutDataTypeStr=boolean
  Relational Operator1 : RelationalOperator  Operator=<  OutDataTypeStr=boolean  RndMeth=Nearest  InputSameDT=on
  Relational Operator2 : RelationalOperator  OutDataTypeStr=boolean  RndMeth=Nearest  InputSameDT=on
  Switch1 : Switch  Criteria=u2 ~= 0  InputSameDT=on
  Switch8 : Switch  Criteria=u2 ~= 0  InputSameDT=on
  Timer_Up : CXLib/Timer_Up
  CEngDsT_stDynTstLck_mp_out : Outport
  wires:
  Constant2/1 -> Timer_Up/3
  Timer_Up/1 -> Relational Operator2/1  "CEngDsT_tiDynTst_mp"
  Constant14/1 -> Timer_Up/1
  Constant1/1 -> Timer_Up/2
  CEngDsT_tiMaxDynTst/1 -> Relational Operator2/2
  Relational Operator2/1 -> Logical Operator1/1
  CEngDsT_t/1 -> Add/1
  CEngDsT_tStrt_mp/1 -> Add/2
  CEngDsT_stRdClnt_mp/1 -> Switch8/2
  Add/1 -> Switch8/1
  Switch8/1 -> Relational Operator1/1, Delay/1  "CEngDsT_dtDynTst_mp"
  Delay/1 -> Switch8/3
  CEngDsT_dtMinDynTst_mp/1 -> Relational Operator1/2
  Relational Operator1/1 -> Logical Operator3/1, Logical Operator1/2
  Logical Operator3/1 -> Logical Operator2/2
  Switch1/1 -> CEngDsT_stDynTstLck_mp_out/1
  Logical Operator1/1 -> Data Type Conversion/1, Logical Operator2/1
  Logical Operator2/1 -> Switch1/2
  Constant3/1 -> Switch1/1
  CEngDsT_stDynTstLck_mp_in/1 -> Switch1/3
  Data Type Conversion/1 -> Data Store Write/1
